simulink model "enabsubs"  (Simulink 6.0)
settings: Solver=ode45  SolverMode=SingleTasking  StartTime=0.0  StopTime=10  MaxStep=0.1  RelTol=1e-3  AbsTol=1e-6
settings Model: Creator=The MathWorks Inc.  LastModifiedBy=batserve  ExtModeTrigMode=oneshot  ExtModeArmWhenConnect=off  ExtModeAutoUpdateStatusClock=off
settings DataIOCC: ExternalInput=[]  InitialState=[]  LimitDataPoints=off
settings OptimizationCC: BooleanDataType=off
settings DebuggingCC: CheckExecutionContextPreStartOutputMsg=on  CheckExecutionContextRuntimeOutputMsg=on  SolverPrmCheckMsg=none
settings HardwareCC: TargetUnknown=on

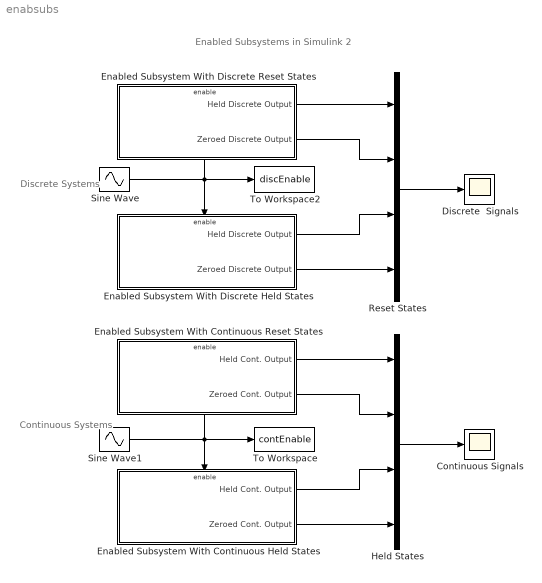
== system enabsubs ==
  note: Enabled Subsystems in Simulink 2
  note: Discrete
      | Systems
  note: Continuous
      | Systems
  Continuous Signals : Scope
      settings: TickLabels=on  SaveName=sys2  DataFormat=Structure
  Discrete  Signals : Scope
      settings: TickLabels=on  SaveName=sys1  DataFormat=Structure
  Enabled Subsystem With Continuous Held States : Subsystem  PropExecContextAcrossSSBoundary=on
  Enabled Subsystem With Continuous Reset States : Subsystem  PropExecContextAcrossSSBoundary=on
  Enabled Subsystem With Discrete Held States : Subsystem  PropExecContextAcrossSSBoundary=on
  Enabled Subsystem With Discrete Reset States : Subsystem  PropExecContextAcrossSSBoundary=on
  Held States : Mux
  Reset States : Mux
  Sine Wave : Sin  Frequency=1/2*pi  SampleTime=0.1
  Sine Wave1 : Sin  Frequency=1/2*pi  SampleTime=0
  To Workspace : ToWorkspace  VariableName=contEnable  SampleTime=-1  SaveFormat=Array
  To Workspace2 : ToWorkspace  VariableName=discEnable  SampleTime=-1  SaveFormat=Array
  wires:
  Enabled Subsystem With Discrete Held States/1(Held Discrete Output) -> Reset States/3
  Enabled Subsystem With Discrete Held States/2(Zeroed Discrete Output) -> Reset States/4
  Enabled Subsystem With Discrete Reset States/1(Held Discrete Output) -> Reset States/1
  Enabled Subsystem With Discrete Reset States/2(Zeroed Discrete Output) -> Reset States/2
  Sine Wave/1 -> Enabled Subsystem With Discrete Held States/Enable, Enabled Subsystem With Discrete Reset States/Enable, To Workspace2/1
  Reset States/1 -> Discrete  Signals/1
  Enabled Subsystem With Continuous Reset States/1(Held Cont. Output) -> Held States/1
  Enabled Subsystem With Continuous Reset States/2(Zeroed Cont. Output) -> Held States/2
  Enabled Subsystem With Continuous Held States/1(Held Cont. Output) -> Held States/3
  Enabled Subsystem With Continuous Held States/2(Zeroed Cont. Output) -> Held States/4
  Sine Wave1/1 -> To Workspace/1, Enabled Subsystem With Continuous Reset States/Enable, Enabled Subsystem With Continuous Held States/Enable
  Held States/1 -> Continuous Signals/1

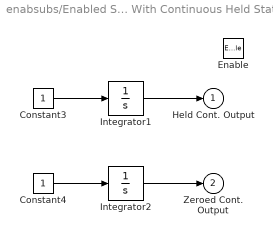
== system enabsubs/Enabled Subsystem With Continuous Held States ==
  Enable : EnablePort
  Constant3 : Constant
  Constant4 : Constant
  Integrator1 : Integrator
  Integrator2 : Integrator
  Held Cont. Output : Outport  InitialOutput=0
  Zeroed Cont. Output : Outport  Port=2  OutputWhenDisabled=reset  InitialOutput=0
  wires:
  Constant3/1 -> Integrator1/1
  Integrator1/1 -> Held Cont. Output/1
  Constant4/1 -> Integrator2/1
  Integrator2/1 -> Zeroed Cont. Output/1

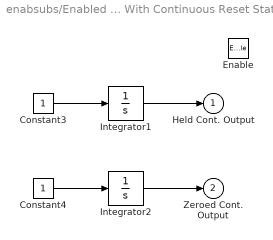
== system enabsubs/Enabled Subsystem With Continuous Reset States ==
  Enable : EnablePort  StatesWhenEnabling=reset
  Constant3 : Constant
  Constant4 : Constant
  Integrator1 : Integrator
  Integrator2 : Integrator
  Held Cont. Output : Outport  InitialOutput=0
  Zeroed Cont. Output : Outport  Port=2  OutputWhenDisabled=reset  InitialOutput=0
  wires:
  Constant3/1 -> Integrator1/1
  Integrator1/1 -> Held Cont. Output/1
  Constant4/1 -> Integrator2/1
  Integrator2/1 -> Zeroed Cont. Output/1

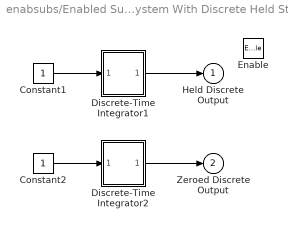
== system enabsubs/Enabled Subsystem With Discrete Held States ==
  Enable : EnablePort
  Constant1 : Constant
  Constant2 : Constant
  Discrete-Time Integrator1 : Subsystem  PropExecContextAcrossSSBoundary=on  mask(Discrete-Time Integrator){@1=0, @2=.1}
      mask prompts: @1 "Initial Condition:"; @2 "Sample Time:"
      mask help: Discrete-Time Integrator:
      mask init:
      | X0=@1;Ts=@2;
      mask Help: Implements a zeroth order discrete\nintegration using a gain, a sum, and\na unit delay. Inputs may be scalar\nor vector.\n
      mask Display: dpoly(Ts,[1 -1],'z')
  Discrete-Time Integrator2 : Subsystem  PropExecContextAcrossSSBoundary=on  mask(Discrete-Time Integrator){@1=0, @2=.1}
      mask prompts: @1 "Initial Condition:"; @2 "Sample Time:"
      mask help: Discrete-Time Integrator:
      mask init:
      | X0=@1;Ts=@2;
      mask Help: Implements a zeroth order discrete\nintegration using a gain, a sum, and\na unit delay. Inputs may be scalar\nor vector.\n
      mask Display: dpoly(Ts,[1 -1],'z')
  Held Discrete Output : Outport  InitialOutput=0
  Zeroed Discrete Output : Outport  Port=2  OutputWhenDisabled=reset  InitialOutput=0
  wires:
  Discrete-Time Integrator2/1(out_1) -> Zeroed Discrete Output/1
  Constant2/1 -> Discrete-Time Integrator2/1(in_1)
  Discrete-Time Integrator1/1(out_1) -> Held Discrete Output/1
  Constant1/1 -> Discrete-Time Integrator1/1(in_1)

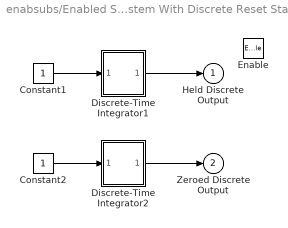
== system enabsubs/Enabled Subsystem With Discrete Reset States ==
  Enable : EnablePort  StatesWhenEnabling=reset
  Constant1 : Constant
  Constant2 : Constant
  Discrete-Time Integrator1 : Subsystem  PropExecContextAcrossSSBoundary=on  mask(Discrete-Time Integrator){@1=0, @2=.1}
      mask prompts: @1 "Initial Condition:"; @2 "Sample Time:"
      mask help: Discrete-Time Integrator:
      mask init:
      | X0=@1;Ts=@2;
      mask Help: Implements a zeroth order discrete\nintegration using a gain, a sum, and\na unit delay. Inputs may be scalar\nor vector.\n
      mask Display: dpoly(Ts,[1 -1],'z')
  Discrete-Time Integrator2 : Subsystem  PropExecContextAcrossSSBoundary=on  mask(Discrete-Time Integrator){@1=0, @2=.1}
      mask prompts: @1 "Initial Condition:"; @2 "Sample Time:"
      mask help: Discrete-Time Integrator:
      mask init:
      | X0=@1;Ts=@2;
      mask Help: Implements a zeroth order discrete\nintegration using a gain, a sum, and\na unit delay. Inputs may be scalar\nor vector.\n
      mask Display: dpoly(Ts,[1 -1],'z')
  Held Discrete Output : Outport  InitialOutput=0
  Zeroed Discrete Output : Outport  Port=2  OutputWhenDisabled=reset  InitialOutput=0
  wires:
  Discrete-Time Integrator2/1(out_1) -> Zeroed Discrete Output/1
  Constant2/1 -> Discrete-Time Integrator2/1(in_1)
  Discrete-Time Integrator1/1(out_1) -> Held Discrete Output/1
  Constant1/1 -> Discrete-Time Integrator1/1(in_1)

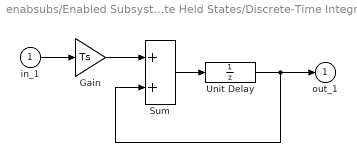
== system enabsubs/Enabled Subsystem With Discrete Held States/Discrete-Time Integrator1 ==
  in_1 : Inport  Port=1  LatchInput=off
  Gain : Gain  Gain=Ts  SaturateOnIntegerOverflow=on
  Sum : Sum  SaturateOnIntegerOverflow=on  InputSameDT=on
  Unit Delay : UnitDelay  X0=X0  SampleTime=Ts
  out_1 : Outport  InitialOutput=0
  wires:
  Unit Delay/1 -> out_1/1, Sum/2
  Sum/1 -> Unit Delay/1
  in_1/1 -> Gain/1
  Gain/1 -> Sum/1

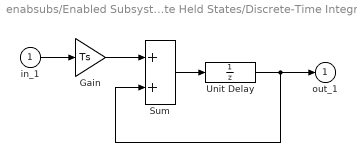
== system enabsubs/Enabled Subsystem With Discrete Held States/Discrete-Time Integrator2 ==
  in_1 : Inport  Port=1  LatchInput=off
  Gain : Gain  Gain=Ts  SaturateOnIntegerOverflow=on
  Sum : Sum  SaturateOnIntegerOverflow=on  InputSameDT=on
  Unit Delay : UnitDelay  X0=X0  SampleTime=Ts
  out_1 : Outport  InitialOutput=0
  wires:
  Unit Delay/1 -> Sum/2, out_1/1
  Sum/1 -> Unit Delay/1
  in_1/1 -> Gain/1
  Gain/1 -> Sum/1

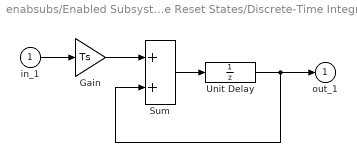
== system enabsubs/Enabled Subsystem With Discrete Reset States/Discrete-Time Integrator1 ==
  in_1 : Inport  Port=1  LatchInput=off
  Gain : Gain  Gain=Ts  SaturateOnIntegerOverflow=on
  Sum : Sum  SaturateOnIntegerOverflow=on  InputSameDT=on
  Unit Delay : UnitDelay  X0=X0  SampleTime=Ts
  out_1 : Outport  InitialOutput=0
  wires:
  Unit Delay/1 -> Sum/2, out_1/1
  Sum/1 -> Unit Delay/1
  in_1/1 -> Gain/1
  Gain/1 -> Sum/1

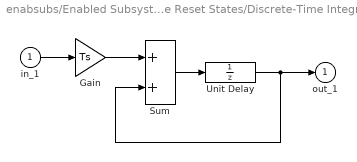
== system enabsubs/Enabled Subsystem With Discrete Reset States/Discrete-Time Integrator2 ==
  in_1 : Inport  Port=1  LatchInput=off
  Gain : Gain  Gain=Ts  SaturateOnIntegerOverflow=on
  Sum : Sum  SaturateOnIntegerOverflow=on  InputSameDT=on
  Unit Delay : UnitDelay  X0=X0  SampleTime=Ts
  out_1 : Outport  InitialOutput=0
  wires:
  Unit Delay/1 -> out_1/1, Sum/2
  Sum/1 -> Unit Delay/1
  in_1/1 -> Gain/1
  Gain/1 -> Sum/1
